simulink model "PertrubeObserve_80400_111_t35"  (R2023b)
settings: Solver=FixedStepAuto  StartTime=0.0  StopTime=3.5  FixedStep=1e-6  RelTol=1e-3
libraries: spsSeriesRLCBranchLib x3, spsDiodeLib x2, spsStairGeneratorLib x2, spsVoltageMeasurementLib x2, spsMosfetLib x1, spsPWMGeneratorDCDCLib x1, spsPVArrayLib x1, spsSeriesRLCLoadLib x1, spspowerguiLib x1
settings Model: Creator=LOUZAZNI  LastModifiedBy=superman-usr
settings SolverCC: AlgebraicLoopSolver=TrustRegion
settings OptimizationCC: ReuseModelBlockBuffer=off
settings DebuggingCC: UnconnectedInputMsg=warning  UnconnectedOutputMsg=warning  UnconnectedLineMsg=warning
settings ModelReferenceCC: EnableRefExpFcnMdlSchedulingChecks=on
settings SFSimCC: CustomCodeUndefinedFunction=UseInterfaceOnly

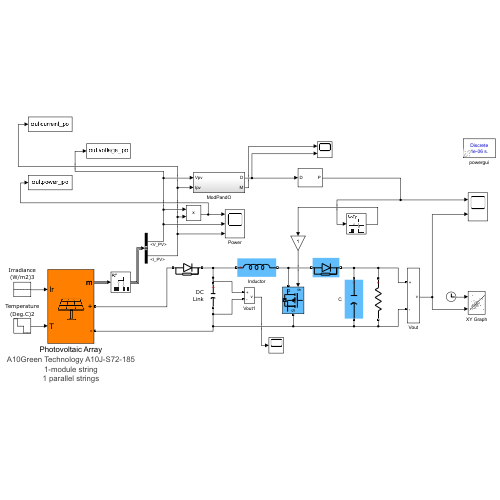
[thumbnail: Simulink's stored preview of the top-level diagram]
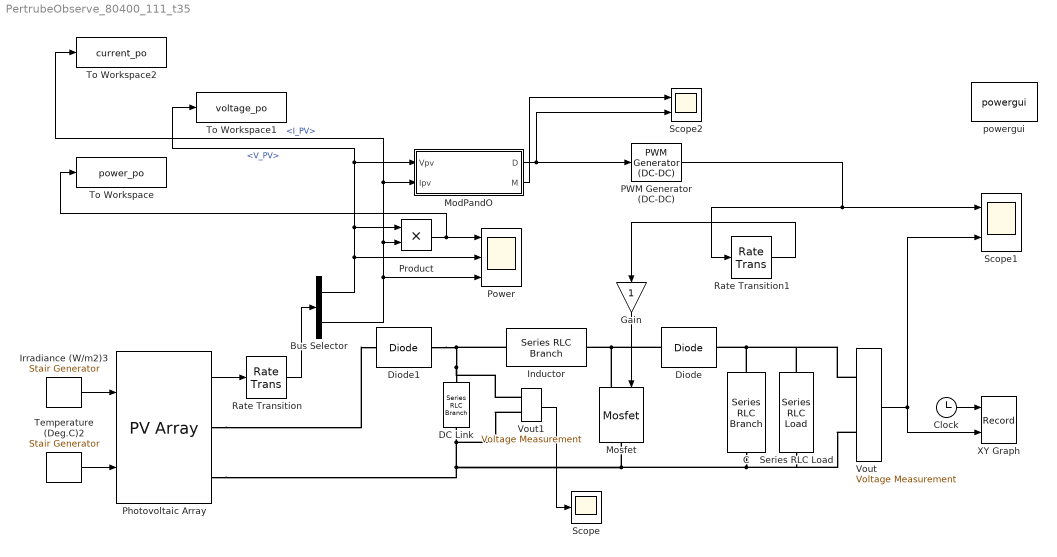
== system PertrubeObserve_80400_111_t35 ==
  Bus Selector : BusSelector  OutputSignals=V_PV,I_PV
  C : spsSeriesRLCBranchLib/Series RLC Branch  LConnTagsString=__new0  RConnTagsString=__new0  BranchType=C  Resistance=1  Inductance=1e-3  SetiL0=off  InitialCurrent=0  Capacitance=50e-6  Setx0=off  InitialVoltage=600  Measurements=None
  Clock : Clock
  DC Link : spsSeriesRLCBranchLib/Series RLC Branch  LConnTagsString=__new0  RConnTagsString=__new0  BranchType=C  Resistance=0.001  Inductance=1.0  SetiL0=off  InitialCurrent=0  Capacitance=4000e-6  Setx0=off  InitialVoltage=310  Measurements=None
  Diode : spsDiodeLib/Diode  Ron=0.001  Lon=0  Vf=0.8  IC=0  UseSnubber=off  Rs=500  Cs=250e-9  Measurements=off
  Diode1 : spsDiodeLib/Diode  Ron=0.001  Lon=0  Vf=0.8  IC=0  UseSnubber=off  Rs=500  Cs=250e-9  Measurements=off
  Gain : Gain
  Inductor : spsSeriesRLCBranchLib/Series RLC Branch  LConnTagsString=__new0  RConnTagsString=__new0  BranchType=L  Resistance=0.01  Inductance=4e-4  SetiL0=off  InitialCurrent=5  Capacitance=1e-6  Setx0=off  InitialVoltage=0  Measurements=None
  Irradiance (W/m2)3 : spsStairGeneratorLib/Stair Generator  t=[0, 0.5, 1, 1.5, 2, 2.5, 3]  e=[1, 1, 1, 1, 1, 1, 1]*1000  Ts=0.0001
  ModPandO : Subsystem
  Mosfet : spsMosfetLib/Mosfet  Ron=0.1  Lon=0  Rd=0.01  Vfd=0  IC=0  Rs=1e5  Cs=inf  Measurements=off
  PWM Generator (DC-DC) : spsPWMGeneratorDCDCLib/PWM Generator (DC-DC)  Fsw=10000  Ts=0
  Photovoltaic Array : spsPVArrayLib/PV Array  Npar=1  Nser=1  PlotType=array @ 1000 W/m2 & specified temperatures  S_vec=[800]  Temp_C_vec=[ 25 ]  ModuleName=A10Green Technology A10J-S72-185  PlotWhenSelected=off  Pm=184.7016  Ncell=72  Voc=44.14  Isc=5.43  Vm=36.72  Im=5.03  beta_Voc_pc=-0.3616  alpha_Isc_pc=0.041492  beta_Voc=-0.15961  alpha_Isc=0.002253  IL=5.4379  I0=1.8755e-10  nI=0.99182  Rsh=257.1494  Rs=0.37471  RobustModel=off  RobustCellTemperature=313.3991  BAL=on  Tc=1e-6  Tfilter=5e-5
      settings: AttributesFormatString=|
      | %<ModuleName>
      | %<Nser>-module string
      | %<Npar> parallel strings
  Power : Scope  NumInputPorts=3
  Product : Product  RndMeth=Zero
  Rate Transition : RateTransition  OutPortSampleTime=1e-6
  Rate Transition1 : RateTransition  OutPortSampleTime=1e-6
  Scope : Scope
  Scope1 : Scope  NumInputPorts=2
  Scope2 : Scope  NumInputPorts=2
  Series RLC Load : spsSeriesRLCLoadLib/Series RLC Load  LConnTagsString=a  RConnTagsString=__new0  NominalVoltage=30  NominalFrequency=50  ActivePower=50  InductivePower=0  CapacitivePower=0  Setx0=off  InitialVoltage=0  SetiL0=off  InitialCurrent=0  Measurements=None  LoadType=constant Z
  Temperature (Deg.C)2 : spsStairGeneratorLib/Stair Generator  t=[0, 0.5, 1, 1.5, 2, 2.5, 3]  e=[80, 80, 40, 40, 0, 0, 0]  Ts=0.0001
  To Workspace : ToWorkspace  VariableName=power_po  SaveFormat=Timeseries  SampleTime=-1
  To Workspace1 : ToWorkspace  VariableName=voltage_po  SaveFormat=Timeseries  SampleTime=-1
  To Workspace2 : ToWorkspace  VariableName=current_po  SaveFormat=Timeseries  SampleTime=-1
  Vout : spsVoltageMeasurementLib/Voltage Measurement  PhasorSimulation=off  OutputType=Complex  PSBequivalent=0
  Vout1 : spsVoltageMeasurementLib/Voltage Measurement  PhasorSimulation=off  OutputType=Complex  PSBequivalent=0
  XY Graph : Record  FileSettingsInternal="{\"entries\":[{\"content\":{\"excelSettings\":{\"content\":{},\"type\":\"Streamout.ExcelSettings\"}},\"type\":\"Streamout.FileSettingStorage\",\"uuid\":\"\"}],\"packageUris\":[\"http:\\/\\/schema.mathworks.com\\/mf0\\/streamout_blocks\\/R2020a\"],\"version\":\"1.0\"}"  Layout=[1 1]  SignalsInternal="{\"entries\":[{\"content\":{\"signals\":[{\"content\":{\"blockPath\":[],\"dimensions\":[1],\"domain\":\"\",\"lineColor\":\"#b746ff\",\"port\":1,\"signalID\":1,\"signalName\":\"Clock\"},\"type\":\"RecordBlkView.Signal\",\"uuid\":\"\"},{\"content\":{\"blockPath\":[],\"dimensions\":[1],\"domain\":\"\",\"lineColor\":\"#64d413\",\"port\":2,\"signalID\":2,\"signalName\":\"Vout\"},\"type\":\"RecordBlkView.Signal\",\"uuid\":\"\"}]},\"type\":\"RecordBlkView.InputSignals\",\"uuid\":\"\"}],\"packageUris\":[\"http:\\/\\/schema.mathworks.com\\/mf0\\/streamout_blocks\\/R2020a\"],\"version\":\"1.0\"}"  VisualizationBindings="{\"xyplotplugin\":{\"info\":[{\"series\":[],\"subplotID\":1}]}}"  CompatibilityTag=XY  st=0.0001
  powergui : spspowerguiLib/powergui  Priority=1  SimulationMode=Discrete  SampleTime=1e-6  frequency=60  Iterations=50  frequencyindice=0  Pbase=100e6  ErrMax=1e-4  UnitsV=kV  UnitsW=MW  buscounter=0  FunctionMessages=off  echomessages=off  EnableUseOfTLC=off  CurrentSourceSwitches=off  DisableSnubberDevices=off  DisableRonSwitches=off  DisableVfSwitches=off  DisplayEquations=off  AutomaticDiscreteSolvers=off  SolverType=Tustin/Backward Euler (TBE)  Interpol=off  ExternalGateDelay=off  methode=off  Ts=100  x0status=blocks  SPID=off  SwTol=0  HookPort=off  NonlinearTolerance=0  nMaxIteration=15  ContinueOnMaxIteration=off  RestoreLinks=warning  ResistiveCurrentMeasurement=off  Frange=[0:2:500]  Ylog=off  Xlog=on  ShowGrid=off  save=off  variable=ZData  structure=0  ZoomFFT=off  StartTime=0.0  cycles=1  DisplayStyle=1  fundamental=60  FreqAxis=off  MaxFrequency=1000  frequencyindicesteady=1  RmsSteady=1  display=off
  wires:
  Vout1/1 -> Scope/1
  Vout/1 -> Scope1/2, XY Graph/2
  Clock/1 -> XY Graph/1
  Bus Selector/1 -> To Workspace1/1, ModPandO/1(Vpv), Product/1, Power/2  "<V_PV>"
  Photovoltaic Array/1 -> Rate Transition/1
  PWM Generator (DC-DC)/1 -> Rate Transition1/1, Scope1/1
  Bus Selector/2 -> ModPandO/2(Ipv), To Workspace2/1, Product/2, Power/3  "<I_PV>"
  Irradiance (W/m2)3/1 -> Photovoltaic Array/1
  Temperature (Deg.C)2/1 -> Photovoltaic Array/2
  ModPandO/1(D) -> PWM Generator (DC-DC)/1, Scope2/2
  Product/1 -> To Workspace/1, Power/1
  ModPandO/2(M) -> Scope2/1
  Gain/1 -> Mosfet/1
  Rate Transition/1 -> Bus Selector/1
  Rate Transition1/1 -> Gain/1
  connections:
  Photovoltaic Array/RConn2 -- Vout1/LConn2 -- DC Link/RConn1 -- Mosfet/RConn1 -- Vout/LConn2 -- Series RLC Load/RConn1 -- C/RConn1
  Mosfet/LConn1 -- Inductor/RConn1 -- Diode/LConn1
  Diode1/RConn1 -- Vout1/LConn1 -- DC Link/LConn1 -- Inductor/LConn1
  C/LConn1 -- Diode/RConn1 -- Vout/LConn1 -- Series RLC Load/LConn1
  Photovoltaic Array/RConn1 -- Diode1/LConn1

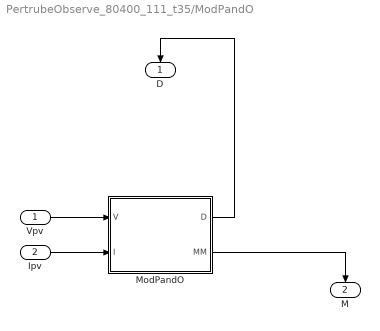
== system PertrubeObserve_80400_111_t35/ModPandO ==
  Vpv : Inport
  Ipv : Inport  Port=2
  ModPandO : MATLAB Function  TreatAsAtomicUnit=on
  D : Outport  VectorParamsAs1DForOutWhenUnconnected=off
  M : Outport  Port=2  VectorParamsAs1DForOutWhenUnconnected=off
  wires:
  ModPandO/1(D) -> D/1
  Vpv/1 -> ModPandO/1(V)
  Ipv/1 -> ModPandO/2(I)
  ModPandO/2(MM) -> M/1

== matlab function PertrubeObserve_80400_111_t35/ModPandO/ModPandO ==
  data: D output; V input; I input; MM output
    function [D, MM ] = ModPandO(V, I)
    
    Dinit = 0.01;  %Initial value for D output
    
    persistent Vold Pold Dold M N;
    
    dataType = 'double';
    
    if isempty(Vold)
        Vold=0;
        Pold=0;
        Dold=Dinit;
        M=1;
        MM=1;
        N=1;
    end
    
    %%
    Ts = 1e-06;
    
    Num1 = 0.2/Ts;
    Num2 = 0.6/Ts;
    Num3 = 1.0/Ts;
    
    deltaD = 0.0005;
    Dmax = 1;      
    Dmin = 0.01;
    
    %%
    noise = 0.1*randn(1);
    P= V*I + noise ;
    dV= V - Vold;
    dP= P - Pold;
    
    N=abs(dP);
    
    if N < 0.0002
        D = Dold;
    else
        if dP < 0
            if dV < 0
                D = Dold - deltaD;
            else
                D = Dold + deltaD;
            end
        else
            if dV < 0
                D = Dold + deltaD;
            else
                D = Dold - deltaD;
            end
        end
    end
    
    
    
    if  D > Dmax
        D = Dmax;
    elseif D < Dmin
        D = Dmin;
    else
        D = D;
    end
    
    %%
    Dold=D;
    Vold=V;
    Pold=P;
    
    M = M+1;
    MM = M;
